simulink model "SimLab3_3"  (R2014b)
settings: Solver=VariableStepAuto  SolverMode=SingleTasking  StartTime=0.0  StopTime=time  RelTol=1e-3
values from neighbouring files (symbols this model uses):
  Amplitude = 20    [Simulations_1.m]    (also in Simulations_2.m = 200; Simulations_2_disc.m; Simulations_3.m; Simulations_4.m)
  Dsp = double(Dsp_d)    [Simulations_4.m]
  Freq = 10    [Simulations_1.m]    (also in Simulations_2.m; Simulations_2_disc.m; Simulations_3.m; Simulations_4.m)
  Isp = double(Isp_d)    [Simulations_4.m]
  L1 = 11.4E-3    (= 0.0114)    [Simulations_1.m]    (also in Simulations_2.m; Simulations_2_disc.m; Simulations_3.m; Simulations_4.m)
  Nsp = double(Nsp_d)    [Simulations_4.m]
  Psp = double(P)    [Simulations_3.m]    (also in Simulations_4.m = double(Psp_d))
  Sine_wave = 1    [Simulations_1.m]    (also in Simulations_2.m; Simulations_2_disc.m; Simulations_3.m; Simulations_4.m)
undefined symbols (not defined in the file or in its folder): Den_FF, dm, Jeq, Kemf, Km, n, Num_FF, pos_ref_step, R
libraries: simulink x1
settings Model: Creator=sofianh  LastModifiedBy=diegogm
settings OptimizationCC: BlockReduction=off  BooleanDataType=off  UseDivisionForNetSlopeComputation=off  SimCompilerOptimization=off
settings DebuggingCC: SaveWithParameterizedLinksMsg=none  UnderspecifiedInitializationDetection=Classic  MergeDetectMultiDrivingBlocksExec=none  SignalResolutionControl=TryResolveAllWithWarning  SolverPrmCheckMsg=none  FrameProcessingCompatibilityMsg=error  AllowSymbolicDim=off
settings HardwareCC: TargetUnknown=on
settings RTWCC: RTWCompilerOptimization=off
settings ConfigComp: CovMetricSettings=dw  CovHtmlReporting=on  CovSaveCumulativeToWorkspaceVar=on  CovSaveSingleToWorkspaceVar=on  CovExternalEMLEnable=off  CovSFcnEnable=off

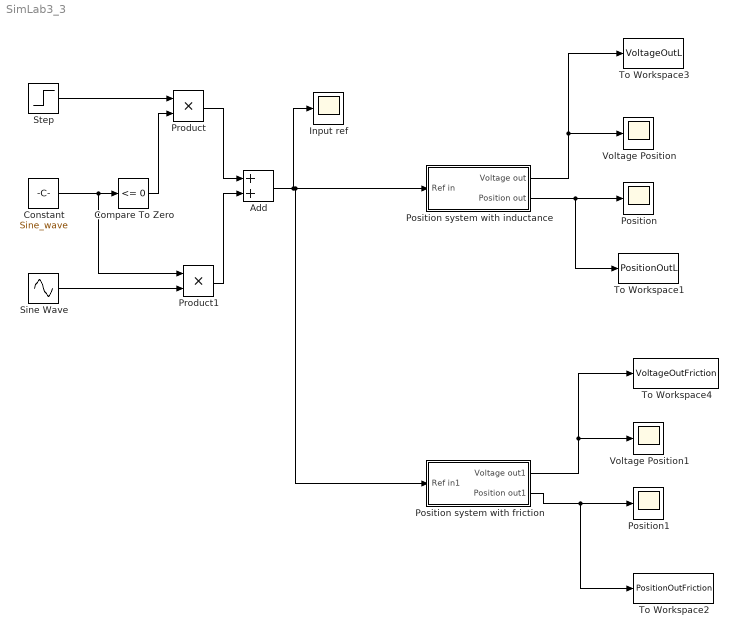
== system SimLab3_3 ==
  Add : Sum
  Compare To Zero : simulink/Logic and Bit Operations/Compare To Zero  relop=<=  OutDataTypeStr=boolean
  Constant : Constant  Value=Sine_wave
  Input ref : Scope
      settings: YMin=10.00000  YMax=30.00000  SaveName=ScopeData6
  Position : Scope
      settings: YMin=-2.652  YMax=23.86797
  Position system with friction : Subsystem
  Position system with inductance : Subsystem
  Position1 : Scope
      settings: YMin=-1.66723  YMax=15.00506
  Product : Product
  Product1 : Product
  Sine Wave : Sin  Amplitude=Amplitude  Frequency=Freq  SampleTime=0
  Step : Step  Time=0  After=pos_ref_step  SampleTime=0
  To Workspace1 : ToWorkspace  VariableName=PositionOutL  SaveFormat=Structure With Time  SampleTime=-1
  To Workspace2 : ToWorkspace  VariableName=PositionOutFriction  SaveFormat=Structure With Time  SampleTime=-1
  To Workspace3 : ToWorkspace  VariableName=VoltageOutL  SaveFormat=Structure With Time  SampleTime=-1
  To Workspace4 : ToWorkspace  VariableName=VoltageOutFriction  SaveFormat=Structure With Time  SampleTime=-1
  Voltage Position : Scope
      settings: YMin=1.38733  YMax=22.06807  SaveName=ScopeData4
  Voltage Position1 : Scope
  wires:
  Position system with inductance/1(Voltage out) -> To Workspace3/1, Voltage Position/1
  Position system with inductance/2(Position out) -> To Workspace1/1, Position/1
  Add/1 -> Position system with friction/1(Ref in1), Position system with inductance/1(Ref in), Input ref/1
  Step/1 -> Product/1
  Constant/1 -> Product1/1, Compare To Zero/1
  Sine Wave/1 -> Product1/2
  Product/1 -> Add/1
  Product1/1 -> Add/2
  Compare To Zero/1 -> Product/2
  Position system with friction/1(Voltage out1) -> To Workspace4/1, Voltage Position1/1
  Position system with friction/2(Position out1) -> To Workspace2/1, Position1/1

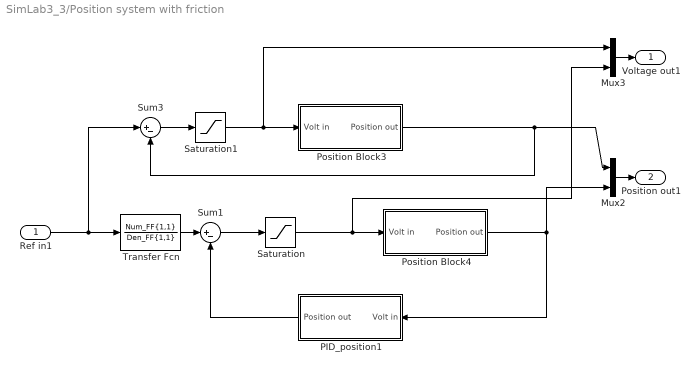
== system SimLab3_3/Position system with friction ==
  Ref in1 : Inport
  Mux2 : Mux  Inputs=2
  Mux3 : Mux  Inputs=2
  PID_position1 : Subsystem
  Position Block3 : Subsystem
  Position Block4 : Subsystem
  Saturation : Saturate  UpperLimit=24  LowerLimit=-24
  Saturation1 : Saturate  UpperLimit=24  LowerLimit=-24
  Sum1 : Sum  Inputs=|+-
  Sum3 : Sum  Inputs=|+-
  Transfer Fcn : TransferFcn  Numerator=Num_FF{1,1}  Denominator=Den_FF{1,1}
  Voltage out1 : Outport
  Position out1 : Outport  Port=2
  wires:
  Position Block4/1(Position out) -> PID_position1/1(Volt in), Mux2/2
  Position Block3/1(Position out) -> Sum3/2, Mux2/1
  Sum3/1 -> Saturation1/1
  Mux2/1 -> Position out1/1
  Mux3/1 -> Voltage out1/1
  Ref in1/1 -> Transfer Fcn/1, Sum3/1
  Sum1/1 -> Saturation/1
  Saturation/1 -> Position Block4/1(Volt in), Mux3/2
  Saturation1/1 -> Position Block3/1(Volt in), Mux3/1
  Transfer Fcn/1 -> Sum1/1
  PID_position1/1(Position out) -> Sum1/2

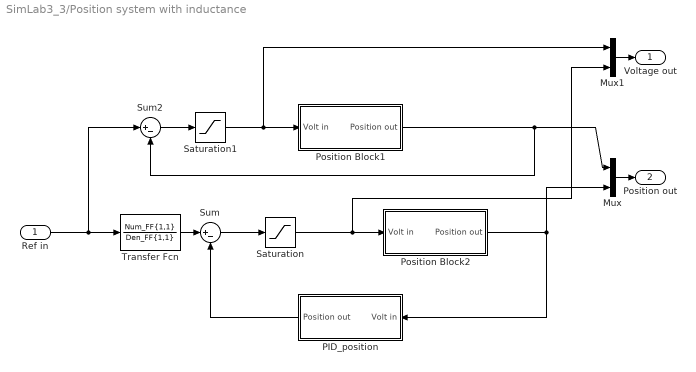
== system SimLab3_3/Position system with inductance ==
  Ref in : Inport
  Mux : Mux  Inputs=2
  Mux1 : Mux  Inputs=2
  PID_position : Subsystem
  Position Block1 : Subsystem
  Position Block2 : Subsystem
  Saturation : Saturate  UpperLimit=24  LowerLimit=-24
  Saturation1 : Saturate  UpperLimit=24  LowerLimit=-24
  Sum : Sum  Inputs=|+-
  Sum2 : Sum  Inputs=|+-
  Transfer Fcn : TransferFcn  Numerator=Num_FF{1,1}  Denominator=Den_FF{1,1}
  Voltage out : Outport
  Position out : Outport  Port=2
  wires:
  Position Block2/1(Position out) -> PID_position/1(Volt in), Mux/2
  Position Block1/1(Position out) -> Sum2/2, Mux/1
  Sum2/1 -> Saturation1/1
  Mux/1 -> Position out/1
  Mux1/1 -> Voltage out/1
  Ref in/1 -> Transfer Fcn/1, Sum2/1
  Sum/1 -> Saturation/1
  Saturation/1 -> Position Block2/1(Volt in), Mux1/2
  Saturation1/1 -> Mux1/1, Position Block1/1(Volt in)
  Transfer Fcn/1 -> Sum/1
  PID_position/1(Position out) -> Sum/2

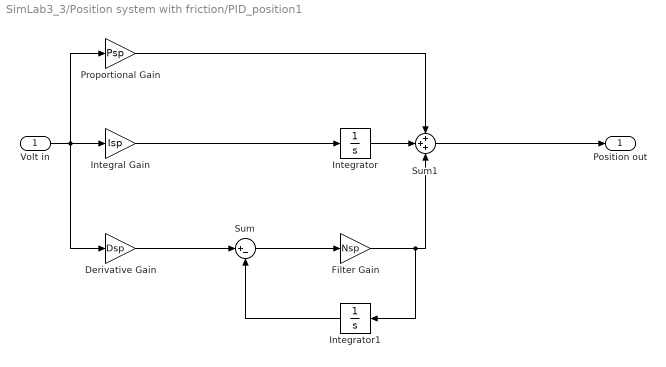
== system SimLab3_3/Position system with friction/PID_position1 ==
  Volt in : Inport
  Derivative Gain : Gain  Gain=Dsp
  Filter Gain : Gain  Gain=Nsp
  Integral Gain : Gain  Gain=Isp
  Integrator : Integrator
  Integrator1 : Integrator
  Proportional Gain : Gain  Gain=Psp
  Sum : Sum  Inputs=|+-
  Sum1 : Sum  Inputs=+++
  Position out : Outport
  wires:
  Sum1/1 -> Position out/1
  Integrator/1 -> Sum1/2
  Integrator1/1 -> Sum/2
  Filter Gain/1 -> Sum1/3, Integrator1/1
  Sum/1 -> Filter Gain/1
  Derivative Gain/1 -> Sum/1
  Integral Gain/1 -> Integrator/1
  Proportional Gain/1 -> Sum1/1
  Volt in/1 -> Derivative Gain/1, Integral Gain/1, Proportional Gain/1

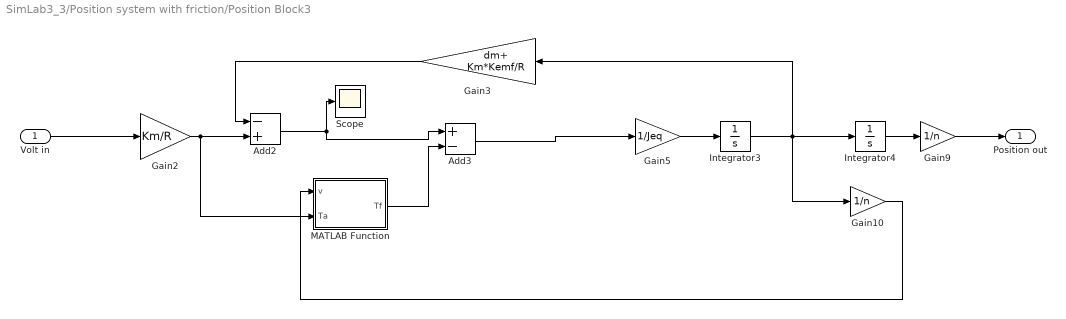
== system SimLab3_3/Position system with friction/Position Block3 ==
  Volt in : Inport
  Add2 : Sum  Inputs=-+
  Add3 : Sum  Inputs=+-
  Gain10 : Gain  Gain=1/n
  Gain2 : Gain  Gain=Km/R
  Gain3 : Gain  Gain=dm+ Km*Kemf/R
  Gain5 : Gain  Gain=1/Jeq
  Gain9 : Gain  Gain=1/n
  Integrator3 : Integrator
  Integrator4 : Integrator
  MATLAB Function : MATLAB Function  TreatAsAtomicUnit=on
  Scope : Scope
      settings: YMin=-10  YMax=10  SaveName=ScopeData2
  Position out : Outport
  wires:
  Gain2/1 -> MATLAB Function/2(Ta), Add2/2
  Gain3/1 -> Add2/1
  Gain5/1 -> Integrator3/1
  Gain10/1 -> MATLAB Function/1(v)
  Volt in/1 -> Gain2/1
  Add3/1 -> Gain5/1
  Add2/1 -> Add3/1, Scope/1
  MATLAB Function/1(Tf) -> Add3/2
  Integrator3/1 -> Integrator4/1, Gain3/1, Gain10/1
  Integrator4/1 -> Gain9/1
  Gain9/1 -> Position out/1

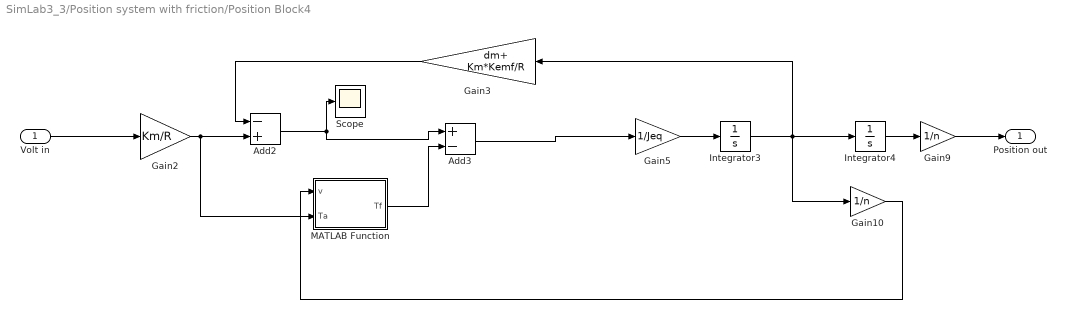
== system SimLab3_3/Position system with friction/Position Block4 ==
  Volt in : Inport
  Add2 : Sum  Inputs=-+
  Add3 : Sum  Inputs=+-
  Gain10 : Gain  Gain=1/n
  Gain2 : Gain  Gain=Km/R
  Gain3 : Gain  Gain=dm+ Km*Kemf/R
  Gain5 : Gain  Gain=1/Jeq
  Gain9 : Gain  Gain=1/n
  Integrator3 : Integrator
  Integrator4 : Integrator
  MATLAB Function : MATLAB Function  TreatAsAtomicUnit=on
  Scope : Scope
      settings: YMin=-10  YMax=10  SaveName=ScopeData2
  Position out : Outport
  wires:
  Gain2/1 -> MATLAB Function/2(Ta), Add2/2
  Gain3/1 -> Add2/1
  Gain5/1 -> Integrator3/1
  Gain10/1 -> MATLAB Function/1(v)
  Volt in/1 -> Gain2/1
  Add3/1 -> Gain5/1
  Add2/1 -> Add3/1, Scope/1
  MATLAB Function/1(Tf) -> Add3/2
  Integrator3/1 -> Integrator4/1, Gain3/1, Gain10/1
  Integrator4/1 -> Gain9/1
  Gain9/1 -> Position out/1

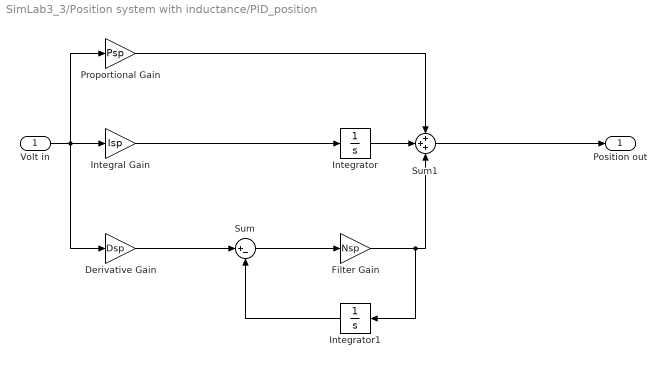
== system SimLab3_3/Position system with inductance/PID_position ==
  Volt in : Inport
  Derivative Gain : Gain  Gain=Dsp
  Filter Gain : Gain  Gain=Nsp
  Integral Gain : Gain  Gain=Isp
  Integrator : Integrator
  Integrator1 : Integrator
  Proportional Gain : Gain  Gain=Psp
  Sum : Sum  Inputs=|+-
  Sum1 : Sum  Inputs=+++
  Position out : Outport
  wires:
  Sum1/1 -> Position out/1
  Integrator/1 -> Sum1/2
  Integrator1/1 -> Sum/2
  Filter Gain/1 -> Sum1/3, Integrator1/1
  Sum/1 -> Filter Gain/1
  Derivative Gain/1 -> Sum/1
  Integral Gain/1 -> Integrator/1
  Proportional Gain/1 -> Sum1/1
  Volt in/1 -> Derivative Gain/1, Integral Gain/1, Proportional Gain/1

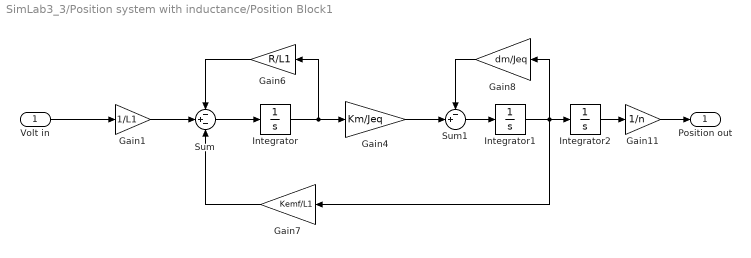
== system SimLab3_3/Position system with inductance/Position Block1 ==
  Volt in : Inport
  Gain1 : Gain  Gain=1/L1
  Gain11 : Gain  Gain=1/n
  Gain4 : Gain  Gain=Km/Jeq
  Gain6 : Gain  Gain=R/L1
  Gain7 : Gain  Gain=Kemf/L1
  Gain8 : Gain  Gain=dm/Jeq
  Integrator : Integrator
  Integrator1 : Integrator
  Integrator2 : Integrator
  Sum : Sum  Inputs=-+-
  Sum1 : Sum  Inputs=-+|
  Position out : Outport
  wires:
  Gain1/1 -> Sum/2
  Sum/1 -> Integrator/1
  Integrator/1 -> Gain6/1, Gain4/1
  Sum1/1 -> Integrator1/1
  Gain4/1 -> Sum1/2
  Integrator1/1 -> Gain8/1, Gain7/1, Integrator2/1
  Gain6/1 -> Sum/1
  Gain7/1 -> Sum/3
  Gain8/1 -> Sum1/1
  Gain11/1 -> Position out/1
  Volt in/1 -> Gain1/1
  Integrator2/1 -> Gain11/1

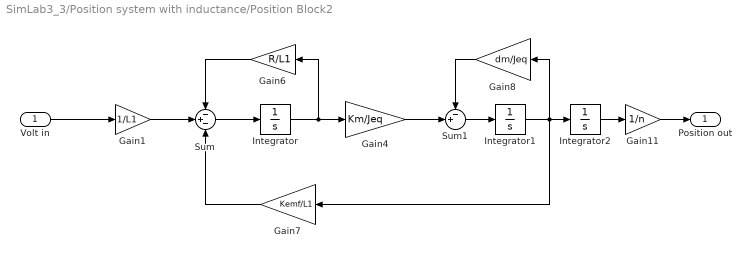
== system SimLab3_3/Position system with inductance/Position Block2 ==
  Volt in : Inport
  Gain1 : Gain  Gain=1/L1
  Gain11 : Gain  Gain=1/n
  Gain4 : Gain  Gain=Km/Jeq
  Gain6 : Gain  Gain=R/L1
  Gain7 : Gain  Gain=Kemf/L1
  Gain8 : Gain  Gain=dm/Jeq
  Integrator : Integrator
  Integrator1 : Integrator
  Integrator2 : Integrator
  Sum : Sum  Inputs=-+-
  Sum1 : Sum  Inputs=-+|
  Position out : Outport
  wires:
  Gain1/1 -> Sum/2
  Sum/1 -> Integrator/1
  Integrator/1 -> Gain6/1, Gain4/1
  Sum1/1 -> Integrator1/1
  Gain4/1 -> Sum1/2
  Integrator1/1 -> Gain8/1, Gain7/1, Integrator2/1
  Gain6/1 -> Sum/1
  Gain7/1 -> Sum/3
  Gain8/1 -> Sum1/1
  Gain11/1 -> Position out/1
  Volt in/1 -> Gain1/1
  Integrator2/1 -> Gain11/1

== matlab function SimLab3_3/Position system with friction/Position Block3/MATLAB Function ==
  data: v input; Tf output; Ta input
function Tf = fcn(v,Ta)
Tc = 1e-3;
dv = 1e-1;
if abs(v) < dv
    if abs(Ta) > Tc
        Tf = Tc*sign(Ta);
    else
        Tf = Ta;
    end
else
    Tf = Tc*sign(v);
end

== matlab function SimLab3_3/Position system with friction/Position Block4/MATLAB Function ==
  data: v input; Tf output; Ta input
function Tf = fcn(v,Ta)
Tc = 1e-3;
dv = 1e-1;
if abs(v) < dv
    if abs(Ta) > Tc
        Tf = Tc*sign(Ta);
    else
        Tf = Ta;
    end
else
    Tf = Tc*sign(v);
end
